simulink library "csu_mpl_mass_properties_mtv_lib"  (R2014b)
settings: Solver=ode45  StartTime=0.0  StopTime=10.0  RelTol=1e-3
undefined symbols (not defined in the file or in its folder): mpl_cg_dry, mpl_gn2_center_tank1, mpl_gn2_center_tank2, mpl_gn2_center_tank3, mpl_gn2_center_tank4, mpl_gn2_center_tank5, mpl_gn2_center_tank6, mpl_gn2_cg_table, mpl_gn2_drain_efficiency_tank1, mpl_gn2_drain_efficiency_tank2, mpl_gn2_drain_efficiency_tank3, mpl_gn2_drain_efficiency_tank4, mpl_gn2_drain_efficiency_tank5, mpl_gn2_drain_efficiency_tank6, mpl_gn2_inertia_table_tank1, mpl_gn2_inertia_table_tank2, mpl_gn2_inertia_table_tank3, mpl_gn2_inertia_table_tank4, mpl_gn2_inertia_table_tank5, mpl_gn2_inertia_table_tank6, mpl_gn2_mass_initial_tank1, mpl_gn2_mass_initial_tank2, mpl_gn2_mass_initial_tank3, mpl_gn2_mass_initial_tank4, mpl_gn2_mass_initial_tank5, mpl_gn2_mass_initial_tank6, mpl_gn2_mass_table, mpl_htp_center_tank1, mpl_htp_center_tank2, mpl_htp_center_tank3, mpl_htp_center_tank4, mpl_htp_cg_table, mpl_htp_drain_efficiency_tank1, mpl_htp_drain_efficiency_tank2, mpl_htp_drain_efficiency_tank3, mpl_htp_drain_efficiency_tank4, mpl_htp_inertia_table_tank1, mpl_htp_inertia_table_tank2, mpl_htp_inertia_table_tank3, mpl_htp_inertia_table_tank4, mpl_htp_mass_initial_tank1, mpl_htp_mass_initial_tank2, mpl_htp_mass_initial_tank3, mpl_htp_mass_initial_tank4, mpl_htp_mass_table, mpl_inertia_dry, mpl_mass_dry
libraries: util_mass_prop_lib x40, simulink x24, util_quat_lib x2, util_common_lib x2, util_info_lib x1
(part 2 of 2)

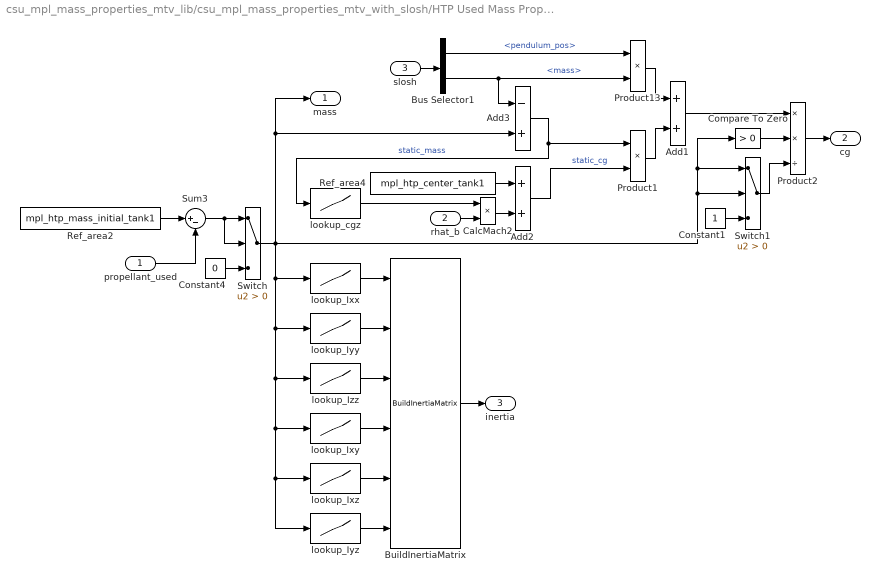
== system csu_mpl_mass_properties_mtv_lib/csu_mpl_mass_properties_mtv_with_slosh/HTP Used Mass Properties1 ==
  propellant_used : Inport
  rhat_b : Inport  Port=2
  slosh : Inport  Port=3
  Add1 : Sum
  Add2 : Sum
  Add3 : Sum  Inputs=-+
  BuildInertiaMatrix : util_mass_prop_lib/BuildInertiaMatrix  SystemSampleTime=-1
  Bus Selector1 : BusSelector  OutputSignals=pendulum_pos,mass
  CalcMach2 : Product  SaturateOnIntegerOverflow=on  OutDataTypeStr=Inherit: Same as first input
  Compare To Zero : simulink/Logic and Bit Operations/Compare To Zero  relop=>  OutDataTypeStr=boolean
  Constant1 : Constant
  Constant4 : Constant  Value=0
  Product1 : Product  SaturateOnIntegerOverflow=on  OutDataTypeStr=Inherit: Same as first input
  Product13 : Product  SaturateOnIntegerOverflow=on  OutDataTypeStr=Inherit: Same as first input
  Product2 : Product  Inputs=**/  SaturateOnIntegerOverflow=on  OutDataTypeStr=Inherit: Same as first input
  Ref_area2 : Constant  Value=mpl_htp_mass_initial_tank1
  Ref_area4 : Constant  Value=mpl_htp_center_tank1
  Sum3 : Sum  Inputs=|+-
  Switch : Switch  Criteria=u2 > Threshold  SaturateOnIntegerOverflow=on
  Switch1 : Switch  Criteria=u2 > Threshold  SaturateOnIntegerOverflow=on
  lookup_Ixx : Lookup  InputValues=mpl_htp_mass_table  Table=mpl_htp_inertia_table_tank1(:,1)
  lookup_Ixy : Lookup  InputValues=mpl_htp_mass_table  Table=mpl_htp_inertia_table_tank1(:,4)
  lookup_Ixz : Lookup  InputValues=mpl_htp_mass_table  Table=mpl_htp_inertia_table_tank1(:,5)
  lookup_Iyy : Lookup  InputValues=mpl_htp_mass_table  Table=mpl_htp_inertia_table_tank1(:,2)
  lookup_Iyz : Lookup  InputValues=mpl_htp_mass_table  Table=mpl_htp_inertia_table_tank1(:,6)
  lookup_Izz : Lookup  InputValues=mpl_htp_mass_table  Table=mpl_htp_inertia_table_tank1(:,3)
  lookup_cgz : Lookup  InputValues=mpl_htp_mass_table  Table=mpl_htp_cg_table(:,3)
  mass : Outport
  cg : Outport  Port=2
  inertia : Outport  Port=3
  wires:
  Compare To Zero/1 -> Product2/2
  Switch1/1 -> Product2/3
  Constant1/1 -> Switch1/3
  Add1/1 -> Product2/1
  Product1/1 -> Add1/2
  Product13/1 -> Add1/1
  Bus Selector1/2 -> Product13/2, Add3/1  "<mass>"
  Bus Selector1/1 -> Product13/1  "<pendulum_pos>"
  Add3/1 -> Product1/1, lookup_cgz/1  "static_mass"
  Product2/1 -> cg/1
  slosh/1 -> Bus Selector1/1
  rhat_b/1 -> CalcMach2/2
  lookup_cgz/1 -> CalcMach2/1
  Constant4/1 -> Switch/3
  Sum3/1 -> Switch/1, Switch/2
  Switch/1 -> lookup_Ixx/1, lookup_Iyy/1, lookup_Izz/1, lookup_Ixy/1, lookup_Ixz/1, lookup_Iyz/1, mass/1, Add3/2, Switch1/2, Switch1/1, Compare To Zero/1
  CalcMach2/1 -> Add2/2
  Ref_area4/1 -> Add2/1
  lookup_Ixx/1 -> BuildInertiaMatrix/1
  lookup_Iyy/1 -> BuildInertiaMatrix/2
  lookup_Izz/1 -> BuildInertiaMatrix/3
  lookup_Ixy/1 -> BuildInertiaMatrix/4
  lookup_Ixz/1 -> BuildInertiaMatrix/5
  lookup_Iyz/1 -> BuildInertiaMatrix/6
  BuildInertiaMatrix/1 -> inertia/1
  Ref_area2/1 -> Sum3/1
  propellant_used/1 -> Sum3/2
  Add2/1 -> Product1/2  "static_cg"

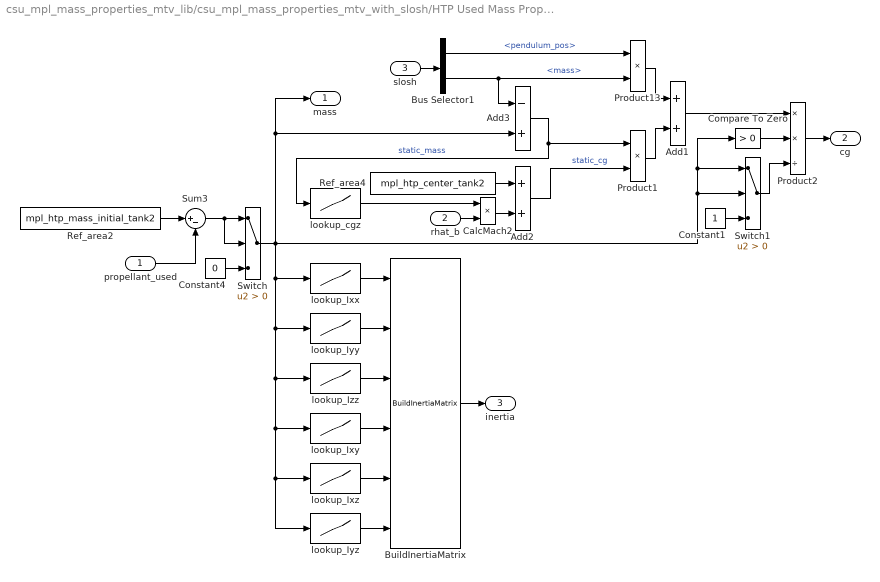
== system csu_mpl_mass_properties_mtv_lib/csu_mpl_mass_properties_mtv_with_slosh/HTP Used Mass Properties2 ==
  propellant_used : Inport
  rhat_b : Inport  Port=2
  slosh : Inport  Port=3
  Add1 : Sum
  Add2 : Sum
  Add3 : Sum  Inputs=-+
  BuildInertiaMatrix : util_mass_prop_lib/BuildInertiaMatrix  SystemSampleTime=-1
  Bus Selector1 : BusSelector  OutputSignals=pendulum_pos,mass
  CalcMach2 : Product  SaturateOnIntegerOverflow=on  OutDataTypeStr=Inherit: Same as first input
  Compare To Zero : simulink/Logic and Bit Operations/Compare To Zero  relop=>  OutDataTypeStr=boolean
  Constant1 : Constant
  Constant4 : Constant  Value=0
  Product1 : Product  SaturateOnIntegerOverflow=on  OutDataTypeStr=Inherit: Same as first input
  Product13 : Product  SaturateOnIntegerOverflow=on  OutDataTypeStr=Inherit: Same as first input
  Product2 : Product  Inputs=**/  SaturateOnIntegerOverflow=on  OutDataTypeStr=Inherit: Same as first input
  Ref_area2 : Constant  Value=mpl_htp_mass_initial_tank2
  Ref_area4 : Constant  Value=mpl_htp_center_tank2
  Sum3 : Sum  Inputs=|+-
  Switch : Switch  Criteria=u2 > Threshold  SaturateOnIntegerOverflow=on
  Switch1 : Switch  Criteria=u2 > Threshold  SaturateOnIntegerOverflow=on
  lookup_Ixx : Lookup  InputValues=mpl_htp_mass_table  Table=mpl_htp_inertia_table_tank2(:,1)
  lookup_Ixy : Lookup  InputValues=mpl_htp_mass_table  Table=mpl_htp_inertia_table_tank2(:,4)
  lookup_Ixz : Lookup  InputValues=mpl_htp_mass_table  Table=mpl_htp_inertia_table_tank2(:,5)
  lookup_Iyy : Lookup  InputValues=mpl_htp_mass_table  Table=mpl_htp_inertia_table_tank2(:,2)
  lookup_Iyz : Lookup  InputValues=mpl_htp_mass_table  Table=mpl_htp_inertia_table_tank2(:,6)
  lookup_Izz : Lookup  InputValues=mpl_htp_mass_table  Table=mpl_htp_inertia_table_tank2(:,3)
  lookup_cgz : Lookup  InputValues=mpl_htp_mass_table  Table=mpl_htp_cg_table(:,3)
  mass : Outport
  cg : Outport  Port=2
  inertia : Outport  Port=3
  wires:
  Compare To Zero/1 -> Product2/2
  Switch1/1 -> Product2/3
  Constant1/1 -> Switch1/3
  Add1/1 -> Product2/1
  Product1/1 -> Add1/2
  Product13/1 -> Add1/1
  Bus Selector1/2 -> Product13/2, Add3/1  "<mass>"
  Bus Selector1/1 -> Product13/1  "<pendulum_pos>"
  Add3/1 -> Product1/1, lookup_cgz/1  "static_mass"
  Product2/1 -> cg/1
  slosh/1 -> Bus Selector1/1
  rhat_b/1 -> CalcMach2/2
  lookup_cgz/1 -> CalcMach2/1
  Constant4/1 -> Switch/3
  Sum3/1 -> Switch/1, Switch/2
  Switch/1 -> lookup_Ixx/1, lookup_Iyy/1, lookup_Izz/1, lookup_Ixy/1, lookup_Ixz/1, lookup_Iyz/1, mass/1, Add3/2, Switch1/2, Switch1/1, Compare To Zero/1
  CalcMach2/1 -> Add2/2
  Ref_area4/1 -> Add2/1
  lookup_Ixx/1 -> BuildInertiaMatrix/1
  lookup_Iyy/1 -> BuildInertiaMatrix/2
  lookup_Izz/1 -> BuildInertiaMatrix/3
  lookup_Ixy/1 -> BuildInertiaMatrix/4
  lookup_Ixz/1 -> BuildInertiaMatrix/5
  lookup_Iyz/1 -> BuildInertiaMatrix/6
  BuildInertiaMatrix/1 -> inertia/1
  Ref_area2/1 -> Sum3/1
  propellant_used/1 -> Sum3/2
  Add2/1 -> Product1/2  "static_cg"

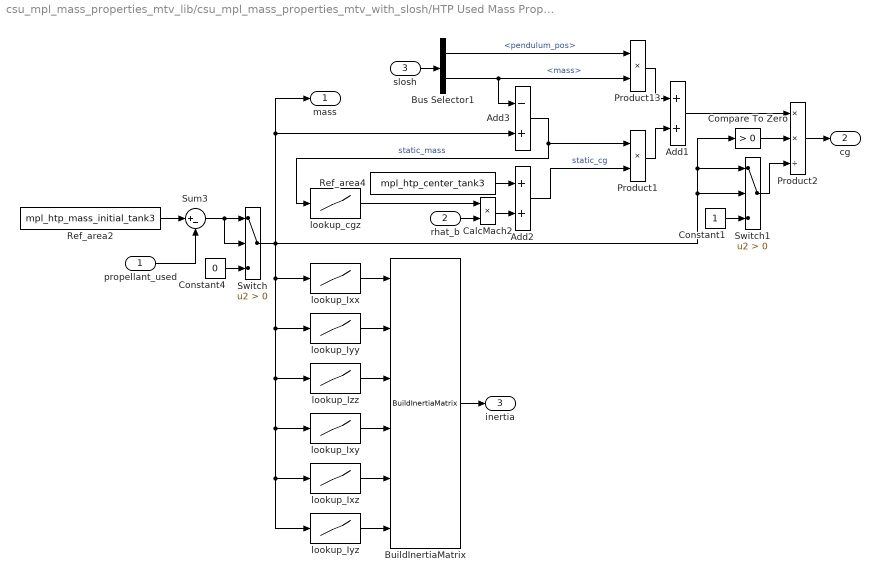
== system csu_mpl_mass_properties_mtv_lib/csu_mpl_mass_properties_mtv_with_slosh/HTP Used Mass Properties3 ==
  propellant_used : Inport
  rhat_b : Inport  Port=2
  slosh : Inport  Port=3
  Add1 : Sum
  Add2 : Sum
  Add3 : Sum  Inputs=-+
  BuildInertiaMatrix : util_mass_prop_lib/BuildInertiaMatrix  SystemSampleTime=-1
  Bus Selector1 : BusSelector  OutputSignals=pendulum_pos,mass
  CalcMach2 : Product  SaturateOnIntegerOverflow=on  OutDataTypeStr=Inherit: Same as first input
  Compare To Zero : simulink/Logic and Bit Operations/Compare To Zero  relop=>  OutDataTypeStr=boolean
  Constant1 : Constant
  Constant4 : Constant  Value=0
  Product1 : Product  SaturateOnIntegerOverflow=on  OutDataTypeStr=Inherit: Same as first input
  Product13 : Product  SaturateOnIntegerOverflow=on  OutDataTypeStr=Inherit: Same as first input
  Product2 : Product  Inputs=**/  SaturateOnIntegerOverflow=on  OutDataTypeStr=Inherit: Same as first input
  Ref_area2 : Constant  Value=mpl_htp_mass_initial_tank3
  Ref_area4 : Constant  Value=mpl_htp_center_tank3
  Sum3 : Sum  Inputs=|+-
  Switch : Switch  Criteria=u2 > Threshold  SaturateOnIntegerOverflow=on
  Switch1 : Switch  Criteria=u2 > Threshold  SaturateOnIntegerOverflow=on
  lookup_Ixx : Lookup  InputValues=mpl_htp_mass_table  Table=mpl_htp_inertia_table_tank3(:,1)
  lookup_Ixy : Lookup  InputValues=mpl_htp_mass_table  Table=mpl_htp_inertia_table_tank3(:,4)
  lookup_Ixz : Lookup  InputValues=mpl_htp_mass_table  Table=mpl_htp_inertia_table_tank3(:,5)
  lookup_Iyy : Lookup  InputValues=mpl_htp_mass_table  Table=mpl_htp_inertia_table_tank3(:,2)
  lookup_Iyz : Lookup  InputValues=mpl_htp_mass_table  Table=mpl_htp_inertia_table_tank3(:,6)
  lookup_Izz : Lookup  InputValues=mpl_htp_mass_table  Table=mpl_htp_inertia_table_tank3(:,3)
  lookup_cgz : Lookup  InputValues=mpl_htp_mass_table  Table=mpl_htp_cg_table(:,3)
  mass : Outport
  cg : Outport  Port=2
  inertia : Outport  Port=3
  wires:
  Compare To Zero/1 -> Product2/2
  Switch1/1 -> Product2/3
  Constant1/1 -> Switch1/3
  Add1/1 -> Product2/1
  Product1/1 -> Add1/2
  Product13/1 -> Add1/1
  Bus Selector1/2 -> Product13/2, Add3/1  "<mass>"
  Bus Selector1/1 -> Product13/1  "<pendulum_pos>"
  Add3/1 -> Product1/1, lookup_cgz/1  "static_mass"
  Product2/1 -> cg/1
  slosh/1 -> Bus Selector1/1
  rhat_b/1 -> CalcMach2/2
  lookup_cgz/1 -> CalcMach2/1
  Constant4/1 -> Switch/3
  Sum3/1 -> Switch/1, Switch/2
  Switch/1 -> lookup_Ixx/1, lookup_Iyy/1, lookup_Izz/1, lookup_Ixy/1, lookup_Ixz/1, lookup_Iyz/1, mass/1, Add3/2, Switch1/2, Switch1/1, Compare To Zero/1
  CalcMach2/1 -> Add2/2
  Ref_area4/1 -> Add2/1
  lookup_Ixx/1 -> BuildInertiaMatrix/1
  lookup_Iyy/1 -> BuildInertiaMatrix/2
  lookup_Izz/1 -> BuildInertiaMatrix/3
  lookup_Ixy/1 -> BuildInertiaMatrix/4
  lookup_Ixz/1 -> BuildInertiaMatrix/5
  lookup_Iyz/1 -> BuildInertiaMatrix/6
  BuildInertiaMatrix/1 -> inertia/1
  Ref_area2/1 -> Sum3/1
  propellant_used/1 -> Sum3/2
  Add2/1 -> Product1/2  "static_cg"

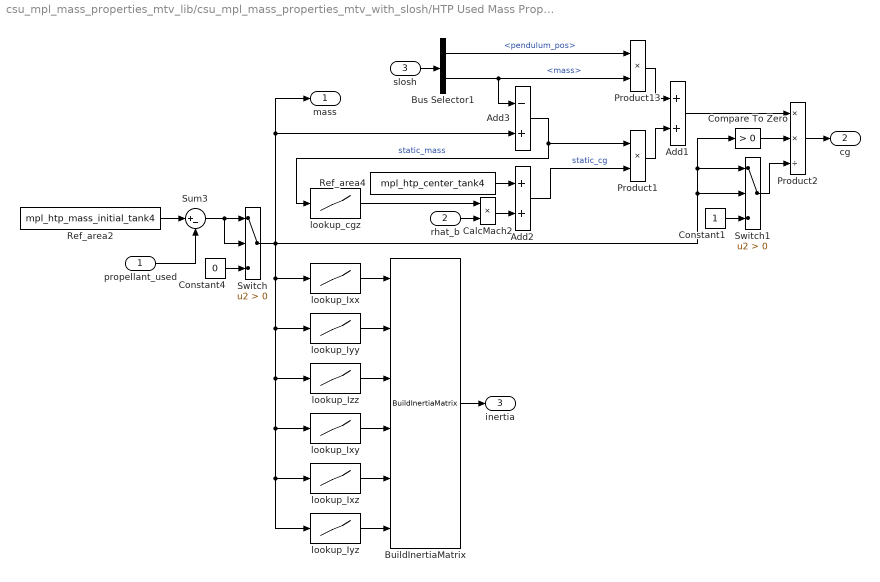
== system csu_mpl_mass_properties_mtv_lib/csu_mpl_mass_properties_mtv_with_slosh/HTP Used Mass Properties4 ==
  propellant_used : Inport
  rhat_b : Inport  Port=2
  slosh : Inport  Port=3
  Add1 : Sum
  Add2 : Sum
  Add3 : Sum  Inputs=-+
  BuildInertiaMatrix : util_mass_prop_lib/BuildInertiaMatrix  SystemSampleTime=-1
  Bus Selector1 : BusSelector  OutputSignals=pendulum_pos,mass
  CalcMach2 : Product  SaturateOnIntegerOverflow=on  OutDataTypeStr=Inherit: Same as first input
  Compare To Zero : simulink/Logic and Bit Operations/Compare To Zero  relop=>  OutDataTypeStr=boolean
  Constant1 : Constant
  Constant4 : Constant  Value=0
  Product1 : Product  SaturateOnIntegerOverflow=on  OutDataTypeStr=Inherit: Same as first input
  Product13 : Product  SaturateOnIntegerOverflow=on  OutDataTypeStr=Inherit: Same as first input
  Product2 : Product  Inputs=**/  SaturateOnIntegerOverflow=on  OutDataTypeStr=Inherit: Same as first input
  Ref_area2 : Constant  Value=mpl_htp_mass_initial_tank4
  Ref_area4 : Constant  Value=mpl_htp_center_tank4
  Sum3 : Sum  Inputs=|+-
  Switch : Switch  Criteria=u2 > Threshold  SaturateOnIntegerOverflow=on
  Switch1 : Switch  Criteria=u2 > Threshold  SaturateOnIntegerOverflow=on
  lookup_Ixx : Lookup  InputValues=mpl_htp_mass_table  Table=mpl_htp_inertia_table_tank4(:,1)
  lookup_Ixy : Lookup  InputValues=mpl_htp_mass_table  Table=mpl_htp_inertia_table_tank4(:,4)
  lookup_Ixz : Lookup  InputValues=mpl_htp_mass_table  Table=mpl_htp_inertia_table_tank4(:,5)
  lookup_Iyy : Lookup  InputValues=mpl_htp_mass_table  Table=mpl_htp_inertia_table_tank4(:,2)
  lookup_Iyz : Lookup  InputValues=mpl_htp_mass_table  Table=mpl_htp_inertia_table_tank4(:,6)
  lookup_Izz : Lookup  InputValues=mpl_htp_mass_table  Table=mpl_htp_inertia_table_tank4(:,3)
  lookup_cgz : Lookup  InputValues=mpl_htp_mass_table  Table=mpl_htp_cg_table(:,3)
  mass : Outport
  cg : Outport  Port=2
  inertia : Outport  Port=3
  wires:
  Compare To Zero/1 -> Product2/2
  Switch1/1 -> Product2/3
  Constant1/1 -> Switch1/3
  Add1/1 -> Product2/1
  Product1/1 -> Add1/2
  Product13/1 -> Add1/1
  Bus Selector1/2 -> Product13/2, Add3/1  "<mass>"
  Bus Selector1/1 -> Product13/1  "<pendulum_pos>"
  Add3/1 -> Product1/1, lookup_cgz/1  "static_mass"
  Product2/1 -> cg/1
  slosh/1 -> Bus Selector1/1
  rhat_b/1 -> CalcMach2/2
  lookup_cgz/1 -> CalcMach2/1
  Constant4/1 -> Switch/3
  Sum3/1 -> Switch/1, Switch/2
  Switch/1 -> lookup_Ixx/1, lookup_Iyy/1, lookup_Izz/1, lookup_Ixy/1, lookup_Ixz/1, lookup_Iyz/1, mass/1, Add3/2, Switch1/2, Switch1/1, Compare To Zero/1
  CalcMach2/1 -> Add2/2
  Ref_area4/1 -> Add2/1
  lookup_Ixx/1 -> BuildInertiaMatrix/1
  lookup_Iyy/1 -> BuildInertiaMatrix/2
  lookup_Izz/1 -> BuildInertiaMatrix/3
  lookup_Ixy/1 -> BuildInertiaMatrix/4
  lookup_Ixz/1 -> BuildInertiaMatrix/5
  lookup_Iyz/1 -> BuildInertiaMatrix/6
  BuildInertiaMatrix/1 -> inertia/1
  Ref_area2/1 -> Sum3/1
  propellant_used/1 -> Sum3/2
  Add2/1 -> Product1/2  "static_cg"

== system csu_mpl_mass_properties_mtv_lib/csu_mpl_mass_properties_mtv_with_slosh/N2 Used Mass Properties1 ==
  propellant_used : Inport
  Add2 : Sum
  BuildInertiaMatrix : util_mass_prop_lib/BuildInertiaMatrix  SystemSampleTime=-1
  Constant4 : Constant  Value=0
  Mux : Mux  Inputs=3
  Ref_area2 : Constant  Value=mpl_gn2_mass_initial_tank1
  Ref_area4 : Constant  Value=mpl_gn2_center_tank1
  Sum3 : Sum  Inputs=|+-
  Switch : Switch  Criteria=u2 > Threshold  SaturateOnIntegerOverflow=on
  lookup_Ixx : Lookup  InputValues=mpl_gn2_mass_table  Table=mpl_gn2_inertia_table_tank1(:,1)
  lookup_Ixy : Lookup  InputValues=mpl_gn2_mass_table  Table=mpl_gn2_inertia_table_tank1(:,4)
  lookup_Ixz : Lookup  InputValues=mpl_gn2_mass_table  Table=mpl_gn2_inertia_table_tank1(:,5)
  lookup_Iyy : Lookup  InputValues=mpl_gn2_mass_table  Table=mpl_gn2_inertia_table_tank1(:,2)
  lookup_Iyz : Lookup  InputValues=mpl_gn2_mass_table  Table=mpl_gn2_inertia_table_tank1(:,6)
  lookup_Izz : Lookup  InputValues=mpl_gn2_mass_table  Table=mpl_gn2_inertia_table_tank1(:,3)
  lookup_cgx : Lookup  InputValues=mpl_gn2_mass_table  Table=mpl_gn2_cg_table(:,1)
  lookup_cgy : Lookup  InputValues=mpl_gn2_mass_table  Table=mpl_gn2_cg_table(:,2)
  lookup_cgz : Lookup  InputValues=mpl_gn2_mass_table  Table=mpl_gn2_cg_table(:,3)
  mass : Outport
  cg : Outport  Port=2
  inertia : Outport  Port=3
  wires:
  Constant4/1 -> Switch/3
  Sum3/1 -> Switch/1, Switch/2
  Switch/1 -> lookup_Iyz/1, lookup_Ixz/1, lookup_Ixy/1, lookup_Izz/1, lookup_Iyy/1, lookup_Ixx/1, lookup_cgz/1, lookup_cgy/1, lookup_cgx/1, mass/1
  Add2/1 -> cg/1
  propellant_used/1 -> Sum3/2
  Ref_area2/1 -> Sum3/1
  lookup_cgx/1 -> Mux/1
  BuildInertiaMatrix/1 -> inertia/1
  lookup_Iyz/1 -> BuildInertiaMatrix/6
  lookup_Ixz/1 -> BuildInertiaMatrix/5
  lookup_Ixy/1 -> BuildInertiaMatrix/4
  lookup_Izz/1 -> BuildInertiaMatrix/3
  lookup_Iyy/1 -> BuildInertiaMatrix/2
  lookup_Ixx/1 -> BuildInertiaMatrix/1
  Ref_area4/1 -> Add2/1
  lookup_cgz/1 -> Mux/3
  lookup_cgy/1 -> Mux/2
  Mux/1 -> Add2/2

== system csu_mpl_mass_properties_mtv_lib/csu_mpl_mass_properties_mtv_with_slosh/N2 Used Mass Properties2 ==
  propellant_used : Inport
  Add2 : Sum
  BuildInertiaMatrix : util_mass_prop_lib/BuildInertiaMatrix  SystemSampleTime=-1
  Constant4 : Constant  Value=0
  Mux : Mux  Inputs=3
  Ref_area2 : Constant  Value=mpl_gn2_mass_initial_tank2
  Ref_area4 : Constant  Value=mpl_gn2_center_tank2
  Sum3 : Sum  Inputs=|+-
  Switch : Switch  Criteria=u2 > Threshold  SaturateOnIntegerOverflow=on
  lookup_Ixx : Lookup  InputValues=mpl_gn2_mass_table  Table=mpl_gn2_inertia_table_tank2(:,1)
  lookup_Ixy : Lookup  InputValues=mpl_gn2_mass_table  Table=mpl_gn2_inertia_table_tank2(:,4)
  lookup_Ixz : Lookup  InputValues=mpl_gn2_mass_table  Table=mpl_gn2_inertia_table_tank2(:,5)
  lookup_Iyy : Lookup  InputValues=mpl_gn2_mass_table  Table=mpl_gn2_inertia_table_tank2(:,2)
  lookup_Iyz : Lookup  InputValues=mpl_gn2_mass_table  Table=mpl_gn2_inertia_table_tank2(:,6)
  lookup_Izz : Lookup  InputValues=mpl_gn2_mass_table  Table=mpl_gn2_inertia_table_tank2(:,3)
  lookup_cgx : Lookup  InputValues=mpl_gn2_mass_table  Table=mpl_gn2_cg_table(:,1)
  lookup_cgy : Lookup  InputValues=mpl_gn2_mass_table  Table=mpl_gn2_cg_table(:,2)
  lookup_cgz : Lookup  InputValues=mpl_gn2_mass_table  Table=mpl_gn2_cg_table(:,3)
  mass : Outport
  cg : Outport  Port=2
  inertia : Outport  Port=3
  wires:
  Constant4/1 -> Switch/3
  Sum3/1 -> Switch/1, Switch/2
  Switch/1 -> lookup_cgx/1, lookup_cgy/1, lookup_cgz/1, lookup_Ixx/1, lookup_Iyy/1, lookup_Izz/1, lookup_Ixy/1, lookup_Ixz/1, lookup_Iyz/1, mass/1
  Mux/1 -> Add2/2
  lookup_cgy/1 -> Mux/2
  lookup_cgz/1 -> Mux/3
  Ref_area4/1 -> Add2/1
  lookup_Ixx/1 -> BuildInertiaMatrix/1
  lookup_Iyy/1 -> BuildInertiaMatrix/2
  lookup_Izz/1 -> BuildInertiaMatrix/3
  lookup_Ixy/1 -> BuildInertiaMatrix/4
  lookup_Ixz/1 -> BuildInertiaMatrix/5
  lookup_Iyz/1 -> BuildInertiaMatrix/6
  BuildInertiaMatrix/1 -> inertia/1
  lookup_cgx/1 -> Mux/1
  Ref_area2/1 -> Sum3/1
  propellant_used/1 -> Sum3/2
  Add2/1 -> cg/1

== system csu_mpl_mass_properties_mtv_lib/csu_mpl_mass_properties_mtv_with_slosh/N2 Used Mass Properties3 ==
  propellant_used : Inport
  Add2 : Sum
  BuildInertiaMatrix : util_mass_prop_lib/BuildInertiaMatrix  SystemSampleTime=-1
  Constant4 : Constant  Value=0
  Mux : Mux  Inputs=3
  Ref_area2 : Constant  Value=mpl_gn2_mass_initial_tank3
  Ref_area4 : Constant  Value=mpl_gn2_center_tank3
  Sum3 : Sum  Inputs=|+-
  Switch : Switch  Criteria=u2 > Threshold  SaturateOnIntegerOverflow=on
  lookup_Ixx : Lookup  InputValues=mpl_gn2_mass_table  Table=mpl_gn2_inertia_table_tank3(:,1)
  lookup_Ixy : Lookup  InputValues=mpl_gn2_mass_table  Table=mpl_gn2_inertia_table_tank3(:,4)
  lookup_Ixz : Lookup  InputValues=mpl_gn2_mass_table  Table=mpl_gn2_inertia_table_tank3(:,5)
  lookup_Iyy : Lookup  InputValues=mpl_gn2_mass_table  Table=mpl_gn2_inertia_table_tank3(:,2)
  lookup_Iyz : Lookup  InputValues=mpl_gn2_mass_table  Table=mpl_gn2_inertia_table_tank3(:,6)
  lookup_Izz : Lookup  InputValues=mpl_gn2_mass_table  Table=mpl_gn2_inertia_table_tank3(:,3)
  lookup_cgx : Lookup  InputValues=mpl_gn2_mass_table  Table=mpl_gn2_cg_table(:,1)
  lookup_cgy : Lookup  InputValues=mpl_gn2_mass_table  Table=mpl_gn2_cg_table(:,2)
  lookup_cgz : Lookup  InputValues=mpl_gn2_mass_table  Table=mpl_gn2_cg_table(:,3)
  mass : Outport
  cg : Outport  Port=2
  inertia : Outport  Port=3
  wires:
  Constant4/1 -> Switch/3
  Sum3/1 -> Switch/1, Switch/2
  Switch/1 -> lookup_cgx/1, mass/1, lookup_Iyz/1, lookup_Ixz/1, lookup_Ixy/1, lookup_Izz/1, lookup_Iyy/1, lookup_Ixx/1, lookup_cgz/1, lookup_cgy/1
  Add2/1 -> cg/1
  propellant_used/1 -> Sum3/2
  Ref_area2/1 -> Sum3/1
  lookup_cgx/1 -> Mux/1
  BuildInertiaMatrix/1 -> inertia/1
  lookup_Iyz/1 -> BuildInertiaMatrix/6
  lookup_Ixz/1 -> BuildInertiaMatrix/5
  lookup_Ixy/1 -> BuildInertiaMatrix/4
  lookup_Izz/1 -> BuildInertiaMatrix/3
  lookup_Iyy/1 -> BuildInertiaMatrix/2
  lookup_Ixx/1 -> BuildInertiaMatrix/1
  Ref_area4/1 -> Add2/1
  lookup_cgz/1 -> Mux/3
  lookup_cgy/1 -> Mux/2
  Mux/1 -> Add2/2

== system csu_mpl_mass_properties_mtv_lib/csu_mpl_mass_properties_mtv_with_slosh/N2 Used Mass Properties4 ==
  propellant_used : Inport
  Add2 : Sum
  BuildInertiaMatrix : util_mass_prop_lib/BuildInertiaMatrix  SystemSampleTime=-1
  Constant4 : Constant  Value=0
  Mux : Mux  Inputs=3
  Ref_area2 : Constant  Value=mpl_gn2_mass_initial_tank4
  Ref_area4 : Constant  Value=mpl_gn2_center_tank4
  Sum3 : Sum  Inputs=|+-
  Switch : Switch  Criteria=u2 > Threshold  SaturateOnIntegerOverflow=on
  lookup_Ixx : Lookup  InputValues=mpl_gn2_mass_table  Table=mpl_gn2_inertia_table_tank4(:,1)
  lookup_Ixy : Lookup  InputValues=mpl_gn2_mass_table  Table=mpl_gn2_inertia_table_tank4(:,4)
  lookup_Ixz : Lookup  InputValues=mpl_gn2_mass_table  Table=mpl_gn2_inertia_table_tank4(:,5)
  lookup_Iyy : Lookup  InputValues=mpl_gn2_mass_table  Table=mpl_gn2_inertia_table_tank4(:,2)
  lookup_Iyz : Lookup  InputValues=mpl_gn2_mass_table  Table=mpl_gn2_inertia_table_tank4(:,6)
  lookup_Izz : Lookup  InputValues=mpl_gn2_mass_table  Table=mpl_gn2_inertia_table_tank4(:,3)
  lookup_cgx : Lookup  InputValues=mpl_gn2_mass_table  Table=mpl_gn2_cg_table(:,1)
  lookup_cgy : Lookup  InputValues=mpl_gn2_mass_table  Table=mpl_gn2_cg_table(:,2)
  lookup_cgz : Lookup  InputValues=mpl_gn2_mass_table  Table=mpl_gn2_cg_table(:,3)
  mass : Outport
  cg : Outport  Port=2
  inertia : Outport  Port=3
  wires:
  Constant4/1 -> Switch/3
  Sum3/1 -> Switch/1, Switch/2
  Switch/1 -> lookup_cgx/1, mass/1, lookup_cgy/1, lookup_cgz/1, lookup_Ixx/1, lookup_Iyy/1, lookup_Izz/1, lookup_Ixy/1, lookup_Ixz/1, lookup_Iyz/1
  Mux/1 -> Add2/2
  lookup_cgy/1 -> Mux/2
  lookup_cgz/1 -> Mux/3
  Ref_area4/1 -> Add2/1
  lookup_Ixx/1 -> BuildInertiaMatrix/1
  lookup_Iyy/1 -> BuildInertiaMatrix/2
  lookup_Izz/1 -> BuildInertiaMatrix/3
  lookup_Ixy/1 -> BuildInertiaMatrix/4
  lookup_Ixz/1 -> BuildInertiaMatrix/5
  lookup_Iyz/1 -> BuildInertiaMatrix/6
  BuildInertiaMatrix/1 -> inertia/1
  lookup_cgx/1 -> Mux/1
  Ref_area2/1 -> Sum3/1
  propellant_used/1 -> Sum3/2
  Add2/1 -> cg/1

== system csu_mpl_mass_properties_mtv_lib/csu_mpl_mass_properties_mtv_with_slosh/N2 Used Mass Properties5 ==
  propellant_used : Inport
  Add2 : Sum
  BuildInertiaMatrix : util_mass_prop_lib/BuildInertiaMatrix  SystemSampleTime=-1
  Constant4 : Constant  Value=0
  Mux : Mux  Inputs=3
  Ref_area2 : Constant  Value=mpl_gn2_mass_initial_tank5
  Ref_area4 : Constant  Value=mpl_gn2_center_tank5
  Sum3 : Sum  Inputs=|+-
  Switch : Switch  Criteria=u2 > Threshold  SaturateOnIntegerOverflow=on
  lookup_Ixx : Lookup  InputValues=mpl_gn2_mass_table  Table=mpl_gn2_inertia_table_tank5(:,1)
  lookup_Ixy : Lookup  InputValues=mpl_gn2_mass_table  Table=mpl_gn2_inertia_table_tank5(:,4)
  lookup_Ixz : Lookup  InputValues=mpl_gn2_mass_table  Table=mpl_gn2_inertia_table_tank5(:,5)
  lookup_Iyy : Lookup  InputValues=mpl_gn2_mass_table  Table=mpl_gn2_inertia_table_tank5(:,2)
  lookup_Iyz : Lookup  InputValues=mpl_gn2_mass_table  Table=mpl_gn2_inertia_table_tank5(:,6)
  lookup_Izz : Lookup  InputValues=mpl_gn2_mass_table  Table=mpl_gn2_inertia_table_tank5(:,3)
  lookup_cgx : Lookup  InputValues=mpl_gn2_mass_table  Table=mpl_gn2_cg_table(:,1)
  lookup_cgy : Lookup  InputValues=mpl_gn2_mass_table  Table=mpl_gn2_cg_table(:,2)
  lookup_cgz : Lookup  InputValues=mpl_gn2_mass_table  Table=mpl_gn2_cg_table(:,3)
  mass : Outport
  cg : Outport  Port=2
  inertia : Outport  Port=3
  wires:
  Constant4/1 -> Switch/3
  Sum3/1 -> Switch/1, Switch/2
  Switch/1 -> lookup_cgx/1, mass/1, lookup_Iyz/1, lookup_Ixz/1, lookup_Ixy/1, lookup_Izz/1, lookup_Iyy/1, lookup_Ixx/1, lookup_cgz/1, lookup_cgy/1
  Add2/1 -> cg/1
  propellant_used/1 -> Sum3/2
  Ref_area2/1 -> Sum3/1
  lookup_cgx/1 -> Mux/1
  BuildInertiaMatrix/1 -> inertia/1
  lookup_Iyz/1 -> BuildInertiaMatrix/6
  lookup_Ixz/1 -> BuildInertiaMatrix/5
  lookup_Ixy/1 -> BuildInertiaMatrix/4
  lookup_Izz/1 -> BuildInertiaMatrix/3
  lookup_Iyy/1 -> BuildInertiaMatrix/2
  lookup_Ixx/1 -> BuildInertiaMatrix/1
  Ref_area4/1 -> Add2/1
  lookup_cgz/1 -> Mux/3
  lookup_cgy/1 -> Mux/2
  Mux/1 -> Add2/2

== system csu_mpl_mass_properties_mtv_lib/csu_mpl_mass_properties_mtv_with_slosh/N2 Used Mass Properties6 ==
  propellant_used : Inport
  Add2 : Sum
  BuildInertiaMatrix : util_mass_prop_lib/BuildInertiaMatrix  SystemSampleTime=-1
  Constant4 : Constant  Value=0
  Mux : Mux  Inputs=3
  Ref_area2 : Constant  Value=mpl_gn2_mass_initial_tank6
  Ref_area4 : Constant  Value=mpl_gn2_center_tank6
  Sum3 : Sum  Inputs=|+-
  Switch : Switch  Criteria=u2 > Threshold  SaturateOnIntegerOverflow=on
  lookup_Ixx : Lookup  InputValues=mpl_gn2_mass_table  Table=mpl_gn2_inertia_table_tank6(:,1)
  lookup_Ixy : Lookup  InputValues=mpl_gn2_mass_table  Table=mpl_gn2_inertia_table_tank6(:,4)
  lookup_Ixz : Lookup  InputValues=mpl_gn2_mass_table  Table=mpl_gn2_inertia_table_tank6(:,5)
  lookup_Iyy : Lookup  InputValues=mpl_gn2_mass_table  Table=mpl_gn2_inertia_table_tank6(:,2)
  lookup_Iyz : Lookup  InputValues=mpl_gn2_mass_table  Table=mpl_gn2_inertia_table_tank6(:,6)
  lookup_Izz : Lookup  InputValues=mpl_gn2_mass_table  Table=mpl_gn2_inertia_table_tank6(:,3)
  lookup_cgx : Lookup  InputValues=mpl_gn2_mass_table  Table=mpl_gn2_cg_table(:,1)
  lookup_cgy : Lookup  InputValues=mpl_gn2_mass_table  Table=mpl_gn2_cg_table(:,2)
  lookup_cgz : Lookup  InputValues=mpl_gn2_mass_table  Table=mpl_gn2_cg_table(:,3)
  mass : Outport
  cg : Outport  Port=2
  inertia : Outport  Port=3
  wires:
  Constant4/1 -> Switch/3
  Sum3/1 -> Switch/1, Switch/2
  Switch/1 -> lookup_cgx/1, lookup_cgy/1, lookup_cgz/1, lookup_Ixx/1, lookup_Iyy/1, lookup_Izz/1, lookup_Ixy/1, lookup_Ixz/1, lookup_Iyz/1, mass/1
  Mux/1 -> Add2/2
  lookup_cgy/1 -> Mux/2
  lookup_cgz/1 -> Mux/3
  Ref_area4/1 -> Add2/1
  lookup_Ixx/1 -> BuildInertiaMatrix/1
  lookup_Iyy/1 -> BuildInertiaMatrix/2
  lookup_Izz/1 -> BuildInertiaMatrix/3
  lookup_Ixy/1 -> BuildInertiaMatrix/4
  lookup_Ixz/1 -> BuildInertiaMatrix/5
  lookup_Iyz/1 -> BuildInertiaMatrix/6
  BuildInertiaMatrix/1 -> inertia/1
  lookup_cgx/1 -> Mux/1
  Ref_area2/1 -> Sum3/1
  propellant_used/1 -> Sum3/2
  Add2/1 -> cg/1

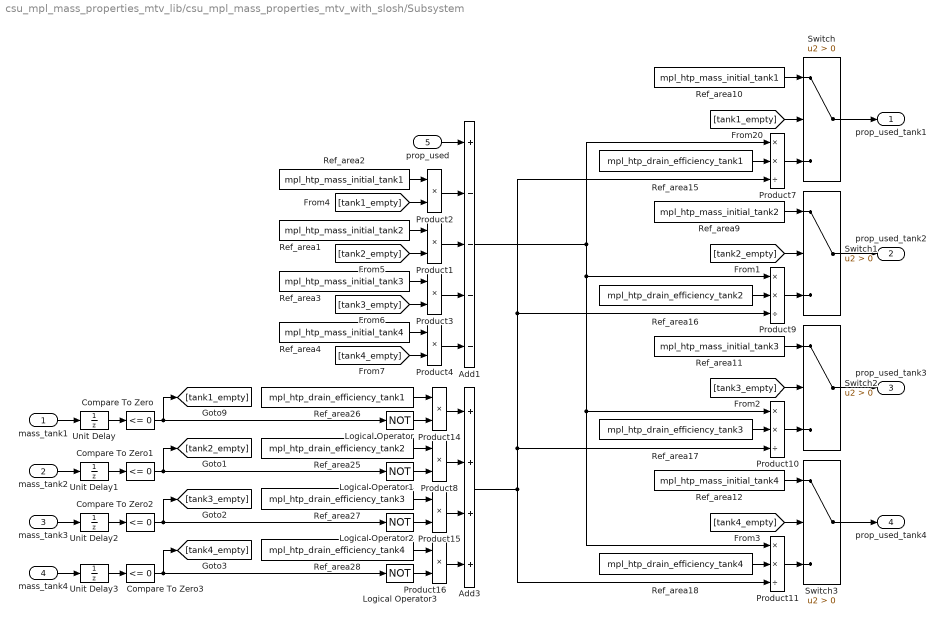
== system csu_mpl_mass_properties_mtv_lib/csu_mpl_mass_properties_mtv_with_slosh/Subsystem ==
  mass_tank1 : Inport
  mass_tank2 : Inport  Port=2
  mass_tank3 : Inport  Port=3
  mass_tank4 : Inport  Port=4
  prop_used : Inport  Port=5
  Add1 : Sum  Inputs=+----  AccumDataTypeStr=double  OutDataTypeStr=double
  Add3 : Sum  Inputs=++++  AccumDataTypeStr=double  OutDataTypeStr=double
  Compare To Zero{,1..3} (4 alike) : simulink/Logic and Bit Operations/Compare To Zero  relop=<=  OutDataTypeStr=boolean
  Logical Operator{,1..3} (4 alike) : Logic  Operator=NOT  AllPortsSameDT=off  OutDataTypeStr=boolean
  Product{1..4,8,14..16} (8 alike) : Product  OutDataTypeStr=double  RndMeth=Zero
  Product{7,9..11} (4 alike) : Product  Inputs=**/  OutDataTypeStr=double  RndMeth=Zero
  Ref_area1 : Constant  Value=mpl_htp_mass_initial_tank2  OutDataTypeStr=double
  Ref_area10 : Constant  Value=mpl_htp_mass_initial_tank1  OutDataTypeStr=double
  Ref_area11 : Constant  Value=mpl_htp_mass_initial_tank3  OutDataTypeStr=double
  Ref_area12 : Constant  Value=mpl_htp_mass_initial_tank4  OutDataTypeStr=double
  Ref_area15 : Constant  Value=mpl_htp_drain_efficiency_tank1  OutDataTypeStr=double
  Ref_area16 : Constant  Value=mpl_htp_drain_efficiency_tank2  OutDataTypeStr=double
  Ref_area17 : Constant  Value=mpl_htp_drain_efficiency_tank3  OutDataTypeStr=double
  Ref_area18 : Constant  Value=mpl_htp_drain_efficiency_tank4  OutDataTypeStr=double
  Ref_area2 : Constant  Value=mpl_htp_mass_initial_tank1  OutDataTypeStr=double
  Ref_area25 : Constant  Value=mpl_htp_drain_efficiency_tank2  OutDataTypeStr=double
  Ref_area26 : Constant  Value=mpl_htp_drain_efficiency_tank1  OutDataTypeStr=double
  Ref_area27 : Constant  Value=mpl_htp_drain_efficiency_tank3  OutDataTypeStr=double
  Ref_area28 : Constant  Value=mpl_htp_drain_efficiency_tank4  OutDataTypeStr=double
  Ref_area3 : Constant  Value=mpl_htp_mass_initial_tank3  OutDataTypeStr=double
  Ref_area4 : Constant  Value=mpl_htp_mass_initial_tank4  OutDataTypeStr=double
  Ref_area9 : Constant  Value=mpl_htp_mass_initial_tank2  OutDataTypeStr=double
  Switch{,1..3} (4 alike) : Switch  Criteria=u2 > Threshold
  Unit Delay : UnitDelay  InitialCondition=mpl_gn2_mass_initial_tank1  SampleTime=-1
  Unit Delay1 : UnitDelay  InitialCondition=mpl_gn2_mass_initial_tank2  SampleTime=-1
  Unit Delay2 : UnitDelay  InitialCondition=mpl_gn2_mass_initial_tank3  SampleTime=-1
  Unit Delay3 : UnitDelay  InitialCondition=mpl_gn2_mass_initial_tank4  SampleTime=-1
  prop_used_tank1 : Outport
  prop_used_tank2 : Outport  Port=2
  prop_used_tank3 : Outport  Port=3
  prop_used_tank4 : Outport  Port=4
  wires:
  Unit Delay3/1 -> Compare To Zero3/1
  Unit Delay2/1 -> Compare To Zero2/1
  Unit Delay1/1 -> Compare To Zero1/1
  Unit Delay/1 -> Compare To Zero/1
  Compare To Zero/1 -> Logical Operator/1, [tank1_empty]
  Compare To Zero3/1 -> Logical Operator3/1, [tank4_empty]
  Compare To Zero2/1 -> Logical Operator2/1, [tank3_empty]
  Compare To Zero1/1 -> Logical Operator1/1, [tank2_empty]
  [tank4_empty] -> Product4/2
  [tank3_empty] -> Product3/2
  [tank2_empty] -> Product1/2
  [tank1_empty] -> Product2/2
  Ref_area4/1 -> Product4/1
  Ref_area3/1 -> Product3/1
  Ref_area1/1 -> Product1/1
  Product1/1 -> Add1/3
  Product3/1 -> Add1/4
  Product4/1 -> Add1/5
  Product2/1 -> Add1/2
  Ref_area2/1 -> Product2/1
  prop_used/1 -> Add1/1
  mass_tank4/1 -> Unit Delay3/1
  mass_tank3/1 -> Unit Delay2/1
  mass_tank2/1 -> Unit Delay1/1
  mass_tank1/1 -> Unit Delay/1
  Ref_area28/1 -> Product16/1
  Ref_area27/1 -> Product15/1
  Ref_area25/1 -> Product8/1
  Ref_area26/1 -> Product14/1
  Product16/1 -> Add3/4
  Product15/1 -> Add3/3
  Product8/1 -> Add3/2
  Product14/1 -> Add3/1
  Logical Operator/1 -> Product14/2
  Logical Operator1/1 -> Product8/2
  Logical Operator2/1 -> Product15/2
  Logical Operator3/1 -> Product16/2
  Ref_area12/1 -> Switch3/1
  [tank4_empty] -> Switch3/2
  Ref_area11/1 -> Switch2/1
  [tank3_empty] -> Switch2/2
  Ref_area9/1 -> Switch1/1
  [tank2_empty] -> Switch1/2
  Ref_area10/1 -> Switch/1
  [tank1_empty] -> Switch/2
  Ref_area15/1 -> Product7/2
  Product7/1 -> Switch/3
  Ref_area16/1 -> Product9/2
  Ref_area17/1 -> Product10/2
  Product10/1 -> Switch2/3
  Product9/1 -> Switch1/3
  Ref_area18/1 -> Product11/2
  Product11/1 -> Switch3/3
  Add1/1 -> Product7/1, Product9/1, Product10/1, Product11/1
  Add3/1 -> Product10/3, Product7/3, Product9/3, Product11/3
  Switch/1 -> prop_used_tank1/1
  Switch1/1 -> prop_used_tank2/1
  Switch2/1 -> prop_used_tank3/1
  Switch3/1 -> prop_used_tank4/1

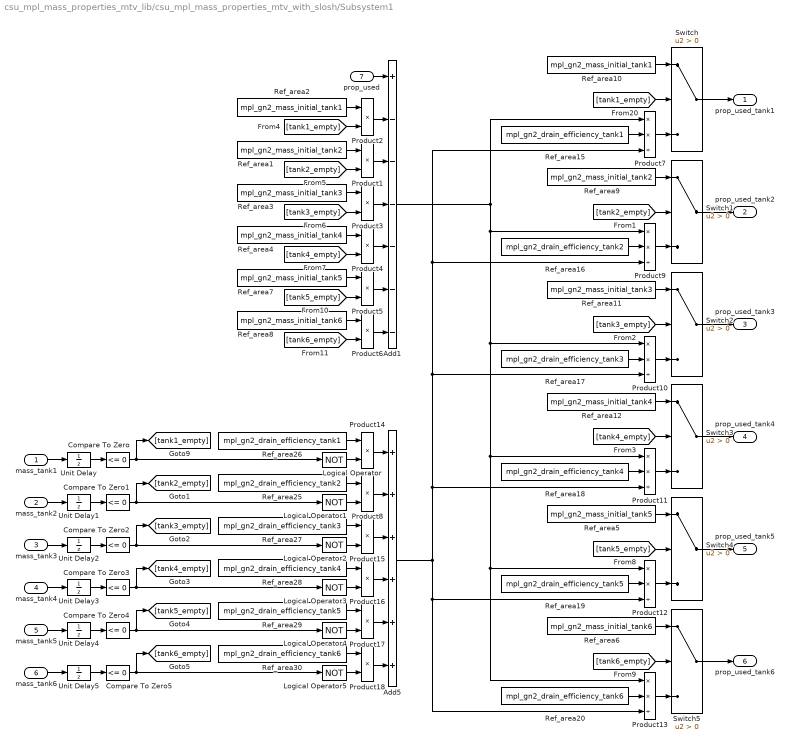
== system csu_mpl_mass_properties_mtv_lib/csu_mpl_mass_properties_mtv_with_slosh/Subsystem1 ==
  mass_tank1 : Inport
  mass_tank2 : Inport  Port=2
  mass_tank3 : Inport  Port=3
  mass_tank4 : Inport  Port=4
  mass_tank5 : Inport  Port=5
  mass_tank6 : Inport  Port=6
  prop_used : Inport  Port=7
  Add1 : Sum  Inputs=+------
  Add5 : Sum  Inputs=++++++  AccumDataTypeStr=double  OutDataTypeStr=double
  Compare To Zero{,1..5} (6 alike) : simulink/Logic and Bit Operations/Compare To Zero  relop=<=  OutDataTypeStr=boolean
  Logical Operator{,1..5} (6 alike) : Logic  Operator=NOT  AllPortsSameDT=off  OutDataTypeStr=boolean
  Product{1..6,8,14..18} (12 alike) : Product  OutDataTypeStr=double  RndMeth=Zero
  Product{7,9..13} (6 alike) : Product  Inputs=**/  OutDataTypeStr=double  RndMeth=Zero
  Ref_area1 : Constant  Value=mpl_gn2_mass_initial_tank2  OutDataTypeStr=double
  Ref_area10 : Constant  Value=mpl_gn2_mass_initial_tank1  OutDataTypeStr=double
  Ref_area11 : Constant  Value=mpl_gn2_mass_initial_tank3  OutDataTypeStr=double
  Ref_area12 : Constant  Value=mpl_gn2_mass_initial_tank4  OutDataTypeStr=double
  Ref_area15 : Constant  Value=mpl_gn2_drain_efficiency_tank1  OutDataTypeStr=double
  Ref_area16 : Constant  Value=mpl_gn2_drain_efficiency_tank2  OutDataTypeStr=double
  Ref_area17 : Constant  Value=mpl_gn2_drain_efficiency_tank3  OutDataTypeStr=double
  Ref_area18 : Constant  Value=mpl_gn2_drain_efficiency_tank4  OutDataTypeStr=double
  Ref_area19 : Constant  Value=mpl_gn2_drain_efficiency_tank5  OutDataTypeStr=double
  Ref_area2 : Constant  Value=mpl_gn2_mass_initial_tank1  OutDataTypeStr=double
  Ref_area20 : Constant  Value=mpl_gn2_drain_efficiency_tank6  OutDataTypeStr=double
  Ref_area25 : Constant  Value=mpl_gn2_drain_efficiency_tank2  OutDataTypeStr=double
  Ref_area26 : Constant  Value=mpl_gn2_drain_efficiency_tank1  OutDataTypeStr=double
  Ref_area27 : Constant  Value=mpl_gn2_drain_efficiency_tank3  OutDataTypeStr=double
  Ref_area28 : Constant  Value=mpl_gn2_drain_efficiency_tank4  OutDataTypeStr=double
  Ref_area29 : Constant  Value=mpl_gn2_drain_efficiency_tank5  OutDataTypeStr=double
  Ref_area3 : Constant  Value=mpl_gn2_mass_initial_tank3  OutDataTypeStr=double
  Ref_area30 : Constant  Value=mpl_gn2_drain_efficiency_tank6  OutDataTypeStr=double
  Ref_area4 : Constant  Value=mpl_gn2_mass_initial_tank4  OutDataTypeStr=double
  Ref_area5 : Constant  Value=mpl_gn2_mass_initial_tank5  OutDataTypeStr=double
  Ref_area6 : Constant  Value=mpl_gn2_mass_initial_tank6  OutDataTypeStr=double
  Ref_area7 : Constant  Value=mpl_gn2_mass_initial_tank5  OutDataTypeStr=double
  Ref_area8 : Constant  Value=mpl_gn2_mass_initial_tank6  OutDataTypeStr=double
  Ref_area9 : Constant  Value=mpl_gn2_mass_initial_tank2  OutDataTypeStr=double
  Switch{,1..5} (6 alike) : Switch  Criteria=u2 > Threshold
  Unit Delay : UnitDelay  InitialCondition=mpl_gn2_mass_initial_tank1  SampleTime=-1
  Unit Delay1 : UnitDelay  InitialCondition=mpl_gn2_mass_initial_tank2  SampleTime=-1
  Unit Delay2 : UnitDelay  InitialCondition=mpl_gn2_mass_initial_tank3  SampleTime=-1
  Unit Delay3 : UnitDelay  InitialCondition=mpl_gn2_mass_initial_tank4  SampleTime=-1
  Unit Delay4 : UnitDelay  InitialCondition=mpl_gn2_mass_initial_tank4  SampleTime=-1
  Unit Delay5 : UnitDelay  InitialCondition=mpl_gn2_mass_initial_tank4  SampleTime=-1
  prop_used_tank1 : Outport
  prop_used_tank2 : Outport  Port=2
  prop_used_tank3 : Outport  Port=3
  prop_used_tank4 : Outport  Port=4
  prop_used_tank5 : Outport  Port=5
  prop_used_tank6 : Outport  Port=6
  wires:
  Unit Delay3/1 -> Compare To Zero3/1
  Unit Delay2/1 -> Compare To Zero2/1
  Unit Delay1/1 -> Compare To Zero1/1
  Unit Delay/1 -> Compare To Zero/1
  Compare To Zero/1 -> [tank1_empty], Logical Operator/1
  Compare To Zero3/1 -> [tank4_empty], Logical Operator3/1
  Compare To Zero2/1 -> [tank3_empty], Logical Operator2/1
  Compare To Zero1/1 -> [tank2_empty], Logical Operator1/1
  [tank4_empty] -> Product4/2
  [tank3_empty] -> Product3/2
  [tank2_empty] -> Product1/2
  [tank1_empty] -> Product2/2
  Ref_area4/1 -> Product4/1
  Ref_area3/1 -> Product3/1
  Ref_area1/1 -> Product1/1
  Product1/1 -> Add1/3
  Product3/1 -> Add1/4
  Product4/1 -> Add1/5
  Product2/1 -> Add1/2
  Ref_area2/1 -> Product2/1
  prop_used/1 -> Add1/1
  mass_tank4/1 -> Unit Delay3/1
  mass_tank3/1 -> Unit Delay2/1
  mass_tank2/1 -> Unit Delay1/1
  mass_tank1/1 -> Unit Delay/1
  Unit Delay4/1 -> Compare To Zero4/1
  Compare To Zero4/1 -> Logical Operator4/1, [tank5_empty]
  mass_tank5/1 -> Unit Delay4/1
  Unit Delay5/1 -> Compare To Zero5/1
  Compare To Zero5/1 -> [tank6_empty], Logical Operator5/1
  mass_tank6/1 -> Unit Delay5/1
  [tank5_empty] -> Product5/2
  Ref_area7/1 -> Product5/1
  [tank6_empty] -> Product6/2
  Ref_area8/1 -> Product6/1
  Product6/1 -> Add1/7
  Product5/1 -> Add1/6
  Ref_area28/1 -> Product16/1
  Ref_area27/1 -> Product15/1
  Ref_area25/1 -> Product8/1
  Ref_area26/1 -> Product14/1
  Ref_area29/1 -> Product17/1
  Ref_area30/1 -> Product18/1
  Product18/1 -> Add5/6
  Product17/1 -> Add5/5
  Product16/1 -> Add5/4
  Product15/1 -> Add5/3
  Product8/1 -> Add5/2
  Product14/1 -> Add5/1
  Logical Operator/1 -> Product14/2
  Logical Operator1/1 -> Product8/2
  Logical Operator2/1 -> Product15/2
  Logical Operator3/1 -> Product16/2
  Logical Operator4/1 -> Product17/2
  Logical Operator5/1 -> Product18/2
  Ref_area12/1 -> Switch3/1
  [tank4_empty] -> Switch3/2
  Ref_area11/1 -> Switch2/1
  [tank3_empty] -> Switch2/2
  Ref_area9/1 -> Switch1/1
  [tank2_empty] -> Switch1/2
  Ref_area10/1 -> Switch/1
  [tank1_empty] -> Switch/2
  Ref_area5/1 -> Switch4/1
  [tank5_empty] -> Switch4/2
  [tank6_empty] -> Switch5/2
  Ref_area6/1 -> Switch5/1
  Ref_area15/1 -> Product7/2
  Product7/1 -> Switch/3
  Ref_area16/1 -> Product9/2
  Ref_area17/1 -> Product10/2
  Product10/1 -> Switch2/3
  Product9/1 -> Switch1/3
  Ref_area18/1 -> Product11/2
  Ref_area19/1 -> Product12/2
  Ref_area20/1 -> Product13/2
  Product13/1 -> Switch5/3
  Product12/1 -> Switch4/3
  Product11/1 -> Switch3/3
  Add1/1 -> Product13/1, Product12/1, Product11/1, Product10/1, Product9/1, Product7/1
  Add5/1 -> Product12/3, Product13/3, Product9/3, Product7/3, Product10/3, Product11/3
  Switch/1 -> prop_used_tank1/1
  Switch1/1 -> prop_used_tank2/1
  Switch2/1 -> prop_used_tank3/1
  Switch3/1 -> prop_used_tank4/1
  Switch4/1 -> prop_used_tank5/1
  Switch5/1 -> prop_used_tank6/1
